simulink model "chap7_7"  (Simulink 3.00)
settings: Solver=ode45  StartTime=0.0  StopTime=20  RelTol=1e-3
libraries: simulink_extras x2

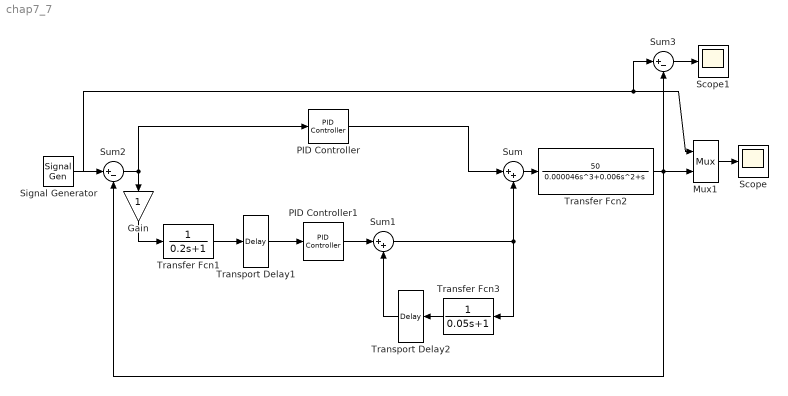
== system chap7_7 ==
  Gain : Gain  Orientation=down  Gain=1  SaturateOnIntegerOverflow=on
  Mux1 : Mux  Inputs=2
      settings: DisplayOption=none
  PID Controller : simulink_extras/Additional Linear/PID Controller  P=1.5  I=30  D=0
  PID Controller1 : simulink_extras/Additional Linear/PID Controller  P=2  I=50  D=0
  Scope : Scope
      settings: TimeRange=auto  YMin=-0.5  YMax=0.55  SaveToWorkspace=off  SaveName=ScopeData  MaxRows=50000
  Scope1 : Scope
      settings: TimeRange=auto  YMin=-0.0009  YMax=0.0006  SaveToWorkspace=off  SaveName=ScopeData  MaxRows=50000
  Signal Generator : SignalGenerator  WaveForm=sine  Amplitude=1  Frequency=0.5  Units=Hertz
  Sum : Sum  Inputs=|++  SaturateOnIntegerOverflow=on
  Sum1 : Sum  Inputs=|++  SaturateOnIntegerOverflow=on
  Sum2 : Sum  Inputs=|+-  SaturateOnIntegerOverflow=on
  Sum3 : Sum  Inputs=|+-  SaturateOnIntegerOverflow=on
  Transfer Fcn1 : TransferFcn  Numerator=[1]  Denominator=[0.2 1]
  Transfer Fcn2 : TransferFcn  Numerator=[50]  Denominator=[0.000046 0.006 1 0]
  Transfer Fcn3 : TransferFcn  Orientation=left  Numerator=[1]  Denominator=[0.05 1]
  Transport Delay1 : TransportDelay  DelayTime=2  InitialInput=0  BufferSize=10240
  Transport Delay2 : TransportDelay  Orientation=left  DelayTime=2  InitialInput=0  BufferSize=10240
  wires:
  Signal Generator/1 -> Sum2/1, Mux1/1, Sum3/1
  Sum2/1 -> PID Controller/1, Gain/1
  Transfer Fcn1/1 -> Transport Delay1/1
  Transport Delay1/1 -> PID Controller1/1
  Transfer Fcn3/1 -> Transport Delay2/1
  Transport Delay2/1 -> Sum1/2
  PID Controller1/1 -> Sum1/1
  Sum/1 -> Transfer Fcn2/1
  PID Controller/1 -> Sum/1
  Sum1/1 -> Transfer Fcn3/1, Sum/2
  Gain/1 -> Transfer Fcn1/1
  Mux1/1 -> Scope/1
  Transfer Fcn2/1 -> Sum2/2, Mux1/2, Sum3/2
  Sum3/1 -> Scope1/1
